simulink model "gm_V1"  (R2017b)
settings: Solver=FixedStepDiscrete  StartTime=0.0  StopTime=Ts_240p*20  RelTol=1e-3
InitFcn:
  | Ts = 1e-3;
  | Ts_240p = 402*324*Ts;
  | Ts_480p = 525*800*Ts;
undefined symbols (not defined in the file or in its folder): gray, Rec, SDTV
libraries: hdlsllib x8, visionhdlio x2, visionconversions x1, visionanalysis x1, visionhdlconversions x1, dspvision x1
settings Model: ModifiedByFormat=The MathWorks Inc.  Creator=The MathWorks, Inc.  LastModifiedBy=The MathWorks Inc.
settings DataIOCC: LimitDataPoints=on  SaveFormat=Array  SaveOutput=off  SaveTime=off
settings OptimizationCC: BlockReduction=off  ConditionallyExecuteInputs=off  DefaultParameterBehavior=Inlined  LifeSpan=inf
settings DebuggingCC: AlgebraicLoopMsg=error  SolverPrmCheckMsg=warning  InheritedTsInSrcMsg=none  SingleTaskRateTransMsg=error  ParameterPrecisionLossMsg=none  AllowSymbolicDim=off  SFUnexpectedBacktrackingDiag=warning  SFNoUnconditionalDefaultTransitionDiag=warning  SFExecutionAtInitializationDiag=none  IntegerSaturationMsg=none
settings HardwareCC: ProdBitPerPointer=32  ProdBitPerSizeT=32  ProdBitPerPtrDiffT=32  ProdLargestAtomicFloat=None  ProdIntDivRoundTo=Undefined  ProdEndianess=Unspecified  ProdWordSize=32  ProdHWDeviceType=ASIC/FPGA->ASIC/FPGA  ProdEqTarget=off
settings ModelReferenceCC: PropagateSignalLabelsOutOfModel=off
settings CodeAppCC: StateflowObjectComments=on
settings GRTTargetCC: TargetLangStandard=C89/C90 (ANSI)  GeneratePreprocessorConditionals=Disable all
settings ConfigComp: CovMetricSettings=dw  CovHtmlReporting=on  CovSaveCumulativeToWorkspaceVar=on  CovSaveSingleToWorkspaceVar=on  CovShowResultsExplorer=off  CovExternalEMLEnable=off  CovSFcnEnable=off

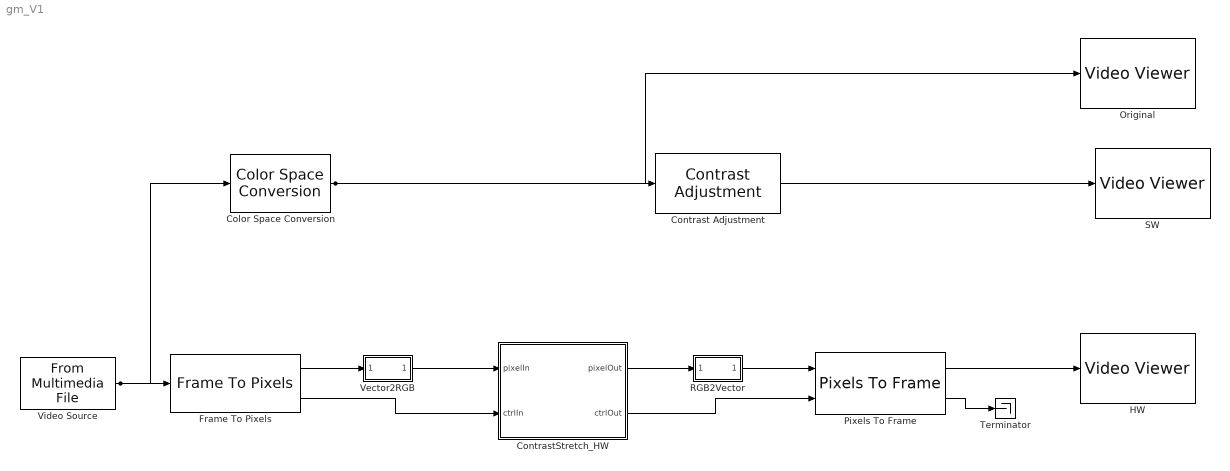
== system gm_V1 ==
  Color Space Conversion : visionconversions/Color Space  Conversion  conversion=Obsolete  conversionActive=R'G'B' to intensity  wp_str=D65  rec=Rec. 601 (SDTV)  sys=1125/60/2:1  imagePorts=One multidimensional signal
      settings: SourceProductName=Computer Vision System Toolbox
  Contrast Adjustment : visionanalysis/Contrast Adjustment  methodInputRange=Range determined by saturating outlier pixels  rangeIn=[0 73]  fracSaturate=[0.5 0.5]  isBinNum=on  binNum=256  methodOutputRange=Full data type range  rangeOut=[0 255]  prod1Mode=Binary point scaling  prod1WordLength=32  prod1FracLength=16  prod2Mode=Binary point scaling  prod2WordLength=32  prod2FracLength=16  roundingMode=Floor  overflowMode=off
      settings: SourceProductName=Computer Vision System Toolbox  SourceProductBaseCode=VP
  ContrastStretch_HW : Subsystem  TreatAsAtomicUnit=on
  Frame To Pixels : visionhdlio/Frame To Pixels  NumComponents=3  VideoFormat=480p  ActivePixelsPerLine=32  ActiveVideoLines=18  TotalPixelsPerLine=42  TotalVideoLines=28  StartingActiveLine=6  FrontPorch=5  SampleTime=0
      settings: SourceProductName=Vision HDL Toolbox  SourceProductBaseCode=VT
  HW : VideoViewer  colormapValue=gray(256)  FigPos=[783.4 735.6 688 514.4]
  Original : VideoViewer  colormapValue=gray(256)  FigPos=[156.2 734.8 688 509.6]
  Pixels To Frame : visionhdlio/Pixels To Frame  NumComponents=3  VideoFormat=480p  ActivePixelsPerLine=32  ActiveVideoLines=18  TotalPixelsPerLine=42  TotalVideoLines=28
      settings: SourceProductName=Vision HDL Toolbox  SourceProductBaseCode=VT
  RGB2Vector : Subsystem
  SW : VideoViewer  colormapValue=gray(256)  FigPos=[309.8 768.4 688 514.4]
  Terminator : Terminator
  Vector2RGB : Subsystem
  Video Source : dspvision/From Multimedia File  inputFilename=E:\RnD\Current_Projects\Musawwir\Frameworks\HW\Musawwir_HW_Zedboard\Custom_IP_Cores\Matlab\ContrastStretching\einstein_bright_640x480.jpg  loop=on  numPlays=inf  outputStreams=Video only  videoDataType=uint8  audioDataType=int16  inheritSampleTime=off  userDefinedSampleTime=Ts_480p  noAudioOutput=off  isIntensityVideo=off  fourcc=RGB  colorVideoFormat=One multidimensional signal  outputEOF=off  dataOrg=Column-major  audioFrameSize=1024  computeAudioFrameSize=off  outSamplingMode=Sample based
      settings: SourceProductBaseCode=VP
  wires:
  Color Space Conversion/1 -> Original/1, Contrast Adjustment/1
  Contrast Adjustment/1 -> SW/1
  ContrastStretch_HW/2(ctrlOut) -> Pixels To Frame/2
  RGB2Vector/1(RGBVector) -> Pixels To Frame/1
  Frame To Pixels/1 -> Vector2RGB/1(RGBVector)
  Frame To Pixels/2 -> ContrastStretch_HW/2(ctrlIn)
  Video Source/1 -> Frame To Pixels/1, Color Space Conversion/1
  ContrastStretch_HW/1(pixelOut) -> RGB2Vector/1(RGB)
  Vector2RGB/1(RGB) -> ContrastStretch_HW/1(pixelIn)
  Pixels To Frame/1 -> HW/1
  Pixels To Frame/2 -> Terminator/1

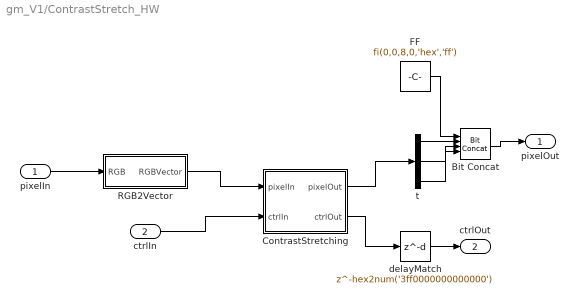
== system gm_V1/ContrastStretch_HW ==
  pixelIn : Inport  OutDataTypeStr=uint32  SampleTime=0.001
  ctrlIn : Inport  Port=2  SampleTime=0.001
  Bit Concat : hdlsllib/Logic and Bit Operations/Bit Concat  numInputs=4
      settings: SourceProductName=HDL Coder  SourceProductBaseCode=HD
  ContrastStretching : Subsystem
  FF : Constant  Value=fi(0,0,8,0,'hex','ff')  OutDataTypeStr=uint8  SampleTime=-1
  RGB2Vector : Subsystem
  delayMatch : Delay  DelayLength=hex2num('3ff0000000000000')  InitialCondition=0  InputProcessing=Inherited  SampleTime=0.001
  t : Demux  Outputs=3
  pixelOut : Outport
  ctrlOut : Outport  Port=2
  wires:
  pixelIn/1 -> RGB2Vector/1(RGB)
  ctrlIn/1 -> ContrastStretching/2(ctrlIn)
  Bit Concat/1 -> pixelOut/1
  ContrastStretching/1(pixelOut) -> t/1
  delayMatch/1 -> ctrlOut/1
  FF/1 -> Bit Concat/1
  RGB2Vector/1(RGBVector) -> ContrastStretching/1(pixelIn)
  t/1 -> Bit Concat/2
  t/2 -> Bit Concat/3
  t/3 -> Bit Concat/4
  ContrastStretching/2(ctrlOut) -> delayMatch/1

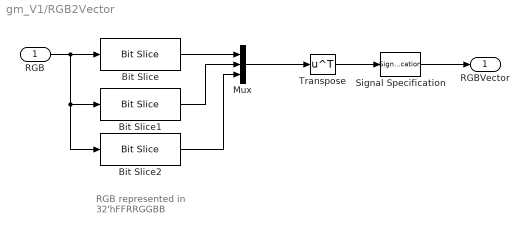
== system gm_V1/RGB2Vector ==
  note: RGB represented in
      | 32'hFFRRGGBB
  RGB : Inport
  Bit Slice : hdlsllib/Logic and Bit Operations/Bit Slice  lidx=23  ridx=16
  Bit Slice1 : hdlsllib/Logic and Bit Operations/Bit Slice  lidx=15  ridx=8
  Bit Slice2 : hdlsllib/Logic and Bit Operations/Bit Slice  lidx=7  ridx=0
  Mux : Mux  Inputs=3
  Signal Specification : SignalSpecification
  Transpose : Math  Operator=transpose  SaturateOnIntegerOverflow=on
  RGBVector : Outport
  wires:
  Signal Specification/1 -> RGBVector/1
  Transpose/1 -> Signal Specification/1
  RGB/1 -> Bit Slice/1, Bit Slice1/1, Bit Slice2/1
  Bit Slice1/1 -> Mux/2
  Bit Slice2/1 -> Mux/3
  Bit Slice/1 -> Mux/1
  Mux/1 -> Transpose/1

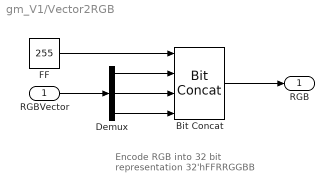
== system gm_V1/Vector2RGB ==
  note: Encode RGB into 32 bit representation
      | 32'hFFRRGGBB
  RGBVector : Inport
  Bit Concat : hdlsllib/Logic and Bit Operations/Bit Concat  numInputs=4
      settings: SourceProductName=HDL Coder  SourceProductBaseCode=HD
  Demux : Demux  Outputs=3
  FF : Constant  Value=255  OutDataTypeStr=uint8  SampleTime=Ts
  RGB : Outport
  wires:
  Demux/3 -> Bit Concat/4
  Demux/2 -> Bit Concat/3
  Demux/1 -> Bit Concat/2
  FF/1 -> Bit Concat/1
  RGBVector/1 -> Demux/1
  Bit Concat/1 -> RGB/1

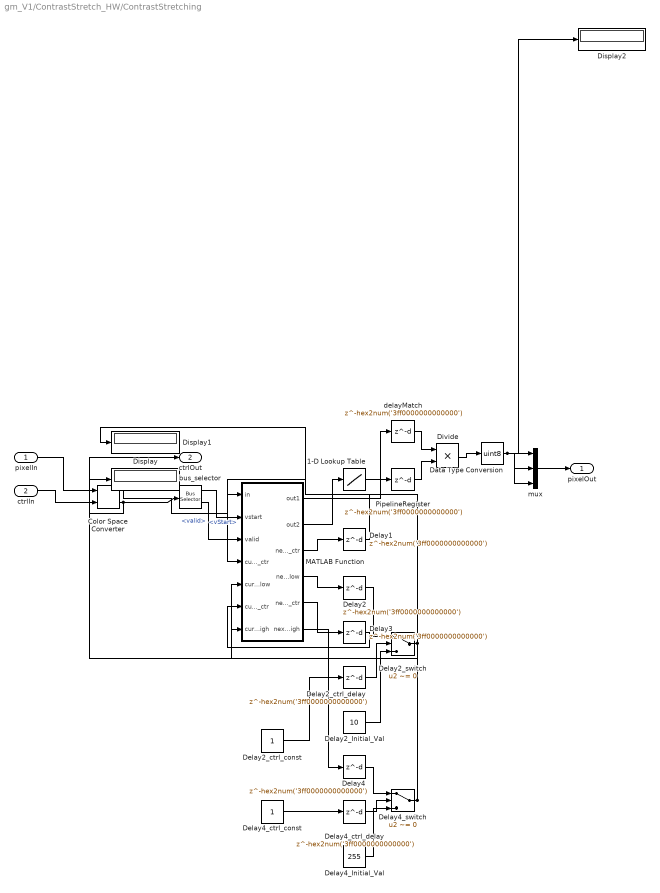
== system gm_V1/ContrastStretch_HW/ContrastStretching ==
  pixelIn : Inport  PortDimensions=3  SampleTime=0.001
  ctrlIn : Inport  Port=2  SampleTime=0.001
  1-D Lookup Table : Lookup_n-D  NumberOfTableDimensions=1  BreakpointsForDimension1=[1 2 3 4 5 6 7 8 9 10 11 12 13 14 15 16 17 18 19 20 21 22 23 24 25 26 27 28 29 30 31 32 33 34 35 36 37 38 39 40 41 42 43 44 45 46 47 48 49 50 51 52 53 54 55 56 57 58 59 60 61 62 63 64 65 66 67 68 69 70 71 72 73 74 75 76 77 78 79 80 81 82 83 84 85 86 87 88 89 90 91 92 93 94 95 96 97 98 99 100 101 102 103 104 105 106 107 108 109 110 111 112 113 114 115 116 117 118 119 120 121 122 123 124 125 126 127 128 129 130 131 132 133 134 135 136 137 138 139 140 141 142 143 144 145 146 147 148 149 150 151 152 153 154 155 156 157 158 159 160 161 162 163 164 165 166 167 168 169 170 171 172 173 174 175 176 177 178 179 180 181 182 183 184 185 186 187 188 189 190 191 192 193 194 195 196 197 198 199 200 201 202 203 204 205 206 207 208 209 210 211 212 213 214 215 216 217 218 219 220 221 222 223 224 225 226 227 228 229 230 231 232 233 234 235 236 237 238 239 240 241 242 243 244 245 246 247 248 249 250 251 252 253 254 255]  Table="reshape([0.999969482421875;0.5;0.333343505859375;0.25;0.20001220703125;0.166656494140625;0.142852783203125;0.125;0.111114501953125;0.100006103515625;0.090911865234375;0.083343505859375;0.076934814453125;0.071441650390625;0.066680908203125;0.0625;0.058837890625;0.0555419921875;0.052642822265625;0.04998779296875;0.047607421875;0.045440673828125;0.043487548828125;0.041656494140625;0.040008544921875;0.0384521484375;0.03704833984375;0.03570556640625;0.03448486328125;0.0333251953125;0.032257080078125;0.03125;0.030303955078125;0.0294189453125;0.028564453125;0.02777099609375;0.02703857421875;0.02630615234375;0.025634765625;0.024993896484375;0.024383544921875;0.0238037109375;0.02325439453125;0.022735595703125;0.022216796875;0.021728515625;0.021270751953125;0.020843505859375;0.020416259765625;0.019989013671875;0.019622802734375;0.01922607421875;0.01885986328125;0.018524169921875;0.0181884765625;0.017852783203125;0.017547607421875;0.017242431640625;0.016937255859375;0.01666259765625;0.016387939453125;0.016143798828125;0.015869140625;0.015625;0.015380859375;0.01513671875;0.014923095703125;0.01470947265625;0.014495849609375;0.0142822265625;0.01409912109375;0.013885498046875;0.013702392578125;0.013519287109375;0.013336181640625;0.013153076171875;0.01300048828125;0.0128173828125;0.012664794921875;0.01251220703125;0.012359619140625;0.01220703125;0.012054443359375;0.01190185546875;0.01177978515625;0.011627197265625;0.011505126953125;0.0113525390625;0.01123046875;0.0111083984375;0.010986328125;0.0108642578125;0.0107421875;0.010650634765625;0.010528564453125;0.010406494140625;0.01031494140625;0.01019287109375;0.010101318359375;0.010009765625;0.0098876953125;0.009796142578125;0.00970458984375;0.009613037109375;0.009521484375;0.009429931640625;0.00933837890625;0.009246826171875;0.009185791015625;0.00909423828125;0.009002685546875;0.008941650390625;0.00885009765625;0.008758544921875;0.008697509765625;0.00860595703125;0.008544921875;0.00848388671875;0.008392333984375;0.008331298828125;0.008270263671875;0.008209228515625;0.00811767578125;0.008056640625;0.00799560546875;0.0079345703125;0.00787353515625;0.0078125;0.00775146484375;0.0076904296875;0.00762939453125;0.007568359375;0.00750732421875;0.007476806640625;0.007415771484375;0.007354736328125;0.007293701171875;0.007232666015625;0.0072021484375;0.00714111328125;0.007080078125;0.007049560546875;0.006988525390625;0.0069580078125;0.00689697265625;0.0068359375;0.006805419921875;0.006744384765625;0.0067138671875;0.00665283203125;0.006622314453125;0.006591796875;0.00653076171875;0.006500244140625;0.006439208984375;0.00640869140625;0.006378173828125;0.006317138671875;0.00628662109375;0.006256103515625;0.0062255859375;0.00616455078125;0.006134033203125;0.006103515625;0.006072998046875;0.006011962890625;0.0059814453125;0.005950927734375;0.00592041015625;0.005889892578125;0.005859375;0.005828857421875;0.005767822265625;0.0057373046875;0.005706787109375;0.00567626953125;0.005645751953125;0.005615234375;0.005584716796875;0.00555419921875;0.005523681640625;0.0054931640625;0.005462646484375;0.00543212890625;0.005401611328125;0.00537109375;0.005340576171875;0.00531005859375;0.005279541015625;0.0052490234375;0.0052490234375;0.005218505859375;0.00518798828125;0.005157470703125;0.005126953125;0.005096435546875;0.00506591796875;0.005035400390625;0.005035400390625;0.0050048828125;0.004974365234375;0.00494384765625;0.004913330078125;0.004913330078125;0.0048828125;0.004852294921875;0.00482177734375;0.00482177734375;0.004791259765625;0.0047607421875;0.004730224609375;0.004730224609375;0.00469970703125;0.004669189453125;0.004638671875;0.004638671875;0.004608154296875;0.00457763671875;0.00457763671875;0.004547119140625;0.0045166015625;0.0045166015625;0.004486083984375;0.00445556640625;0.00445556640625;0.004425048828125;0.00439453125;0.00439453125;0.004364013671875;0.00433349609375;0.00433349609375;0.004302978515625;0.004302978515625;0.0042724609375;0.004241943359375;0.004241943359375;0.00421142578125;0.00421142578125;0.004180908203125;0.004180908203125;0.004150390625;0.004119873046875;0.004119873046875;0.00408935546875;0.00408935546875;0.004058837890625;0.004058837890625;0.0040283203125;0.0040283203125;0.003997802734375;0.003997802734375;0.00396728515625;0.00396728515625;0.003936767578125;0.003936767578125], [1  255])"  InterpMethod=Flat  DiagnosticForOutOfRangeInput=Error  SampleTime=0.001  OutDataTypeStr=fixdt(1, 16, 15)  RndMeth=Simplest  InputSameDT=on
  Color Space Converter : visionhdlconversions/Color Space Converter  Conversion=RGB to intensity  ConversionStandard=Rec. 601 (SDTV)  ScanningStandard=1250/50/2:1  SimulateUsing=Code generation
      settings: SourceProductName=Vision HDL Toolbox  SourceProductBaseCode=VT
  Data Type Conversion : DataTypeConversion  OutDataTypeStr=uint8  SampleTime=0.001
  Delay{1..4} (4 alike) : Delay  DelayLength=hex2num('3ff0000000000000')  InitialCondition=0  InputProcessing=Inherited  SampleTime=0.001
  Delay2_Initial_Val : Constant  Value=10  OutDataTypeStr=uint8  SampleTime=-1
  Delay2_ctrl_const : Constant  OutDataTypeStr=boolean  SampleTime=0.001
  Delay2_ctrl_delay : Delay  DelayLength=hex2num('3ff0000000000000')  InitialCondition=0  InputProcessing=Inherited  SampleTime=0.001
  Delay2_switch : Switch  Criteria=u2 ~= 0  Threshold=hex2num('0000000000000000')  OutDataTypeStr=uint8  SampleTime=0.001
  Delay4_Initial_Val : Constant  Value=255  OutDataTypeStr=uint8  SampleTime=-1
  Delay4_ctrl_const : Constant  OutDataTypeStr=boolean  SampleTime=0.001
  Delay4_ctrl_delay : Delay  DelayLength=hex2num('3ff0000000000000')  InitialCondition=0  InputProcessing=Inherited  SampleTime=0.001
  Delay4_switch : Switch  Criteria=u2 ~= 0  Threshold=hex2num('0000000000000000')  OutDataTypeStr=uint8  SampleTime=0.001
  Display : Display
  Display1 : Display
  Display2 : Display
  Divide : Product  Inputs=**  OutDataTypeStr=fixdt(1, 34, 15)  SampleTime=0.001  SaturateOnIntegerOverflow=on  RndMeth=Zero
  MATLAB Function : Subsystem
  PipelineRegister : Delay  DelayLength=hex2num('3ff0000000000000')  InitialCondition=0  InputProcessing=Inherited  SampleTime=0.001
  bus_selector : BusSelector  OutputSignals=vStart,valid
  delayMatch : Delay  DelayLength=hex2num('3ff0000000000000')  InitialCondition=0  InputProcessing=Inherited  SampleTime=0.001
  mux : Mux  Inputs=3
  pixelOut : Outport
  ctrlOut : Outport  Port=2
  wires:
  PipelineRegister/1 -> Divide/2
  bus_selector/1 -> MATLAB Function/2(vstart)  "<vStart>"
  bus_selector/2 -> MATLAB Function/3(valid)  "<valid>"
  Color Space Converter/1 -> MATLAB Function/1(in)
  Color Space Converter/2 -> bus_selector/1, ctrlOut/1
  Data Type Conversion/1 -> mux/3, mux/2, mux/1, Display2/1
  Delay2_switch/1 -> Display1/1, MATLAB Function/5(curr_low)
  Delay4_switch/1 -> Display/1, MATLAB Function/7(curr_high)
  Divide/1 -> Data Type Conversion/1
  delayMatch/1 -> Divide/1
  MATLAB Function/2(out2) -> 1-D Lookup Table/1
  mux/1 -> pixelOut/1
  Delay2_Initial_Val/1 -> Delay2_switch/3
  Delay2_ctrl_const/1 -> Delay2_ctrl_delay/1
  Delay2_ctrl_delay/1 -> Delay2_switch/2
  Delay4_Initial_Val/1 -> Delay4_switch/3
  Delay4_ctrl_const/1 -> Delay4_ctrl_delay/1
  Delay4_ctrl_delay/1 -> Delay4_switch/2
  pixelIn/1 -> Color Space Converter/1
  ctrlIn/1 -> Color Space Converter/2
  MATLAB Function/1(out1) -> delayMatch/1
  Delay4/1 -> Delay4_switch/1
  Delay3/1 -> MATLAB Function/6(curr_high_ctr)
  Delay2/1 -> Delay2_switch/1
  Delay1/1 -> MATLAB Function/4(curr_low_ctr)
  MATLAB Function/3(next_low_ctr) -> Delay1/1
  MATLAB Function/4(next_low) -> Delay2/1
  MATLAB Function/5(next_high_ctr) -> Delay3/1
  MATLAB Function/6(next_high) -> Delay4/1
  1-D Lookup Table/1 -> PipelineRegister/1

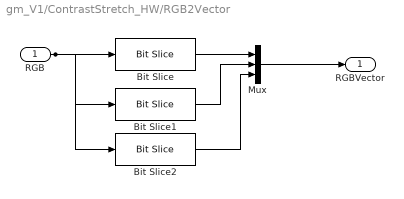
== system gm_V1/ContrastStretch_HW/RGB2Vector ==
  RGB : Inport  SampleTime=0.001
  Bit Slice : hdlsllib/Logic and Bit Operations/Bit Slice  lidx=23  ridx=16
  Bit Slice1 : hdlsllib/Logic and Bit Operations/Bit Slice  lidx=15  ridx=8
  Bit Slice2 : hdlsllib/Logic and Bit Operations/Bit Slice  lidx=7  ridx=0
  Mux : Mux  Inputs=3
  RGBVector : Outport
  wires:
  Bit Slice/1 -> Mux/1
  Bit Slice1/1 -> Mux/2
  Bit Slice2/1 -> Mux/3
  Mux/1 -> RGBVector/1
  RGB/1 -> Bit Slice2/1, Bit Slice1/1, Bit Slice/1

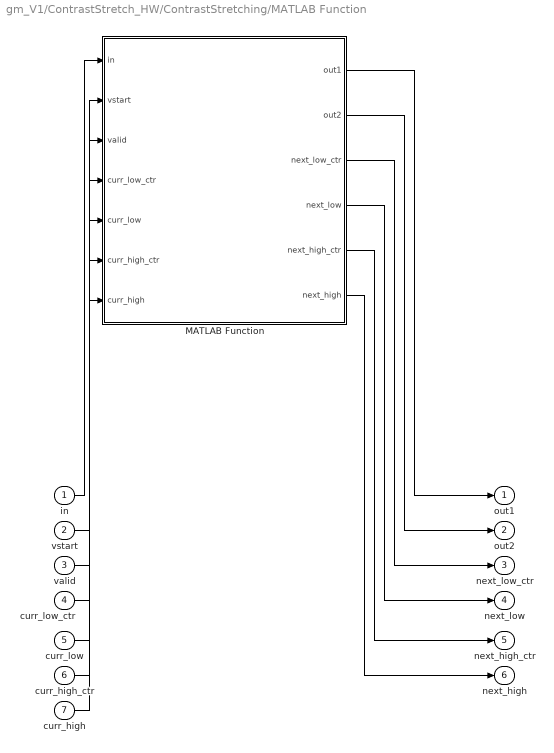
== system gm_V1/ContrastStretch_HW/ContrastStretching/MATLAB Function ==
  in : Inport  SampleTime=0.001
  vstart : Inport  Port=2  SampleTime=0.001
  valid : Inport  Port=3  SampleTime=0.001
  curr_low_ctr : Inport  Port=4  SampleTime=0.001
  curr_low : Inport  Port=5  SampleTime=0.001
  curr_high_ctr : Inport  Port=6  SampleTime=0.001
  curr_high : Inport  Port=7  SampleTime=0.001
  MATLAB Function : MATLAB Function  TreatAsAtomicUnit=on
  out1 : Outport
  out2 : Outport  Port=2
  next_low_ctr : Outport  Port=3
  next_low : Outport  Port=4
  next_high_ctr : Outport  Port=5
  next_high : Outport  Port=6
  wires:
  in/1 -> MATLAB Function/1(in)
  vstart/1 -> MATLAB Function/2(vstart)
  valid/1 -> MATLAB Function/3(valid)
  curr_low_ctr/1 -> MATLAB Function/4(curr_low_ctr)
  curr_low/1 -> MATLAB Function/5(curr_low)
  curr_high_ctr/1 -> MATLAB Function/6(curr_high_ctr)
  curr_high/1 -> MATLAB Function/7(curr_high)
  MATLAB Function/1(out1) -> out1/1
  MATLAB Function/2(out2) -> out2/1
  MATLAB Function/3(next_low_ctr) -> next_low_ctr/1
  MATLAB Function/4(next_low) -> next_low/1
  MATLAB Function/5(next_high_ctr) -> next_high_ctr/1
  MATLAB Function/6(next_high) -> next_high/1

== matlab function gm_V1/ContrastStretch_HW/ContrastStretching/MATLAB Function/MATLAB Function ==
  data: in input; vstart input; valid input; out1 output fixdt(0,18,0) size=[1,1]; out2 output fixdt(0,8,0); curr_low_ctr input fixdt(0,20,0); next_low_ctr output fixdt(0,20,0); curr_low input fixdt(0,8,0); next_low output fixdt(0,8,0); curr_high_ctr input fixdt(0,20,0); curr_high input fixdt(0,8,0); next_high_ctr output fixdt(0,20,0); next_high output fixdt(0,8,0)
function [out1, out2, next_low_ctr, next_low, next_high_ctr, next_high] = lower_limt(in, vstart, valid, curr_low_ctr, curr_low, curr_high_ctr, curr_high)

prob_limit = 2*(320*240)/100;
step = 1;

if(vstart==1)
    next_low_ctr = fi(0,0,20,0);
else
    if((in<curr_low)&(valid==1))
        next_low_ctr = fi(curr_low_ctr + 1,0,20,0);
    else
        next_low_ctr = curr_low_ctr;
    end
end

if(vstart==1)
    if(curr_low_ctr<=prob_limit)%150*curr_low)
        next_low = fi(curr_low + step,0,8,0);
    else
%         if(curr_low>0)
            next_low = fi(curr_low - step,0,8,0);
%         else
%             next_low = curr_low;
%         end
    end
else
    next_low = curr_low;
end

if(vstart==1)
    next_high_ctr = fi(0,0,20,0);
else
    if((in>curr_high)&(valid==1))
        next_high_ctr = fi(curr_high_ctr + 1,0,20,0);
    else
        next_high_ctr = curr_high_ctr;
    end
end

if(vstart==1)
    if(curr_high_ctr<=prob_limit)%150*(255-curr_high))
        next_high = fi(curr_high - step,0,8,0);
    else
%         if(curr_low>0)
            next_high = fi(curr_high + step,0,8,0);
%         else
%             next_low = curr_low;
%         end
    end
else
    next_high = curr_high;
end


low = curr_low;
high = curr_high;
out1 = fi((in-low)*255,0,18,0);
out2 = fi((high-low),0,8,0);
